simulink model "motor_OpenLoopResp"  (R2022b)
settings: Solver=VariableStepAuto  StartTime=0.0  StopTime=5.5  FixedStep=0.001  RelTol=1e-3
values from neighbouring files (symbols this model uses):
  B = 1.413e-05    [parameters_10.4volt.mat]
  J = 3.3e-06    [parameters_10.4volt.mat]
  Kb = 0.0448    [parameters_10.4volt.mat]
  Kt = 0.0412    [parameters_10.4volt.mat]
  La = 0.0534    [parameters_10.4volt.mat]
  Ra = 30    [parameters_10.4volt.mat]
settings Model: Creator=user  LastModifiedBy=chu80
settings DebuggingCC: UnconnectedInputMsg=warning  UnconnectedOutputMsg=warning  UnconnectedLineMsg=warning
settings ModelReferenceCC: EnableRefExpFcnMdlSchedulingChecks=on
settings RTWCC: DLArmComputeVersion=19.05

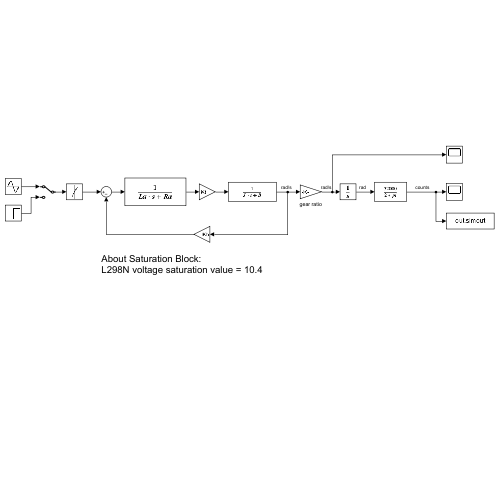
[thumbnail: Simulink's stored preview of the top-level diagram]
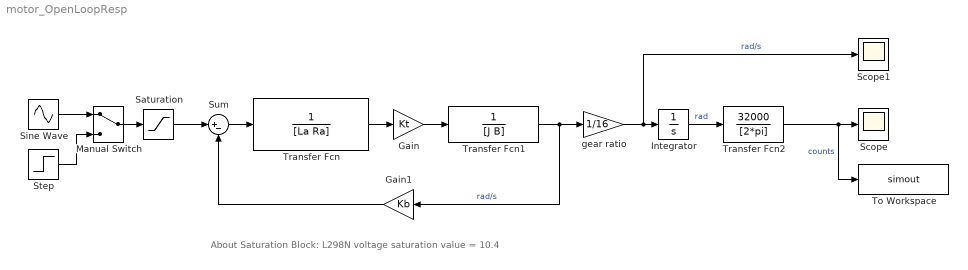
== system motor_OpenLoopResp ==
  note: About Saturation Block:
      | L298N voltage saturation value = 10.4
  Gain : Gain  Gain=Kt
  Gain1 : Gain  Gain=Kb
  Integrator : Integrator
  Manual Switch : ManualSwitch
  Saturation : Saturate  UpperLimit=10.4  LowerLimit=-10.4
  Scope : Scope
  Scope1 : Scope
  Sine Wave : Sin  Amplitude=8.1  Frequency=pi  SampleTime=0
  Step : Step  After=8.1  SampleTime=0
  Sum : Sum  Inputs=|+-
  To Workspace : ToWorkspace  VariableName=simout  SaveFormat=Timeseries  SampleTime=-1
  Transfer Fcn : TransferFcn  Denominator=[La Ra]
  Transfer Fcn1 : TransferFcn  Denominator=[J B]
  Transfer Fcn2 : TransferFcn  Numerator=[32000]  Denominator=[2*pi]
  gear ratio : Gain  Gain=1/16
  wires:
  Transfer Fcn/1 -> Gain/1
  Gain/1 -> Transfer Fcn1/1
  Transfer Fcn1/1 -> gear ratio/1, Gain1/1  "rad/s"
  Sum/1 -> Transfer Fcn/1
  Gain1/1 -> Sum/2
  Integrator/1 -> Transfer Fcn2/1  "rad"
  Transfer Fcn2/1 -> To Workspace/1, Scope/1  "counts"
  Saturation/1 -> Sum/1
  gear ratio/1 -> Scope1/1, Integrator/1  "rad/s"
  Manual Switch/1 -> Saturation/1
  Sine Wave/1 -> Manual Switch/1
  Step/1 -> Manual Switch/2
